simulink model "BF_analyse"  (R2021b)
settings: Solver=VariableStepAuto  StartTime=0.0  StopTime=10.0  RelTol=1e-3
values from neighbouring files (symbols this model uses):
  A = [0 0 0  1 0 0   0 0 0   0 0 0 ... (first row only)    [systune_gain_scheduling.m]    (also in systune_variable_gain_scheduling_LPV.m)
  B = [0 0 0 0 ... (first row only)    [systune_gain_scheduling.m]    (also in systune_variable_gain_scheduling_LPV.m)
  B2 = [0 0 ... (first row only)    [systune_gain_scheduling.m]    (also in systune_variable_gain_scheduling_LPV.m)
  C = eye(12)    [systune_gain_scheduling.m]    (also in systune_variable_gain_scheduling_LPV.m)
  C_control = [1 0 0 0 0 0 0 0 0 1 0 0 ... (96 elements, 8x12)]    [matrix_systune.mat]    (also in systune_gain_scheduling.m = [C(1:7,:);C(9,:)]; systune_variable_gain_scheduling_LPV.m = [C(1:7,:);C(9:12,:)])
  D = zeros(12,6)    [systune_gain_scheduling.m]    (also in systune_variable_gain_scheduling_LPV.m)
  F = [1  0; 1  0; 0  1; 0  1]    [matrix_systune.mat]    (also in systune_gain_scheduling.m = [1 0; 1 0; 0 1; 0 1]; systune_variable_gain_scheduling_LPV.m = [1 0; 1 0; 0 1; 0 1])
  H_val = [-3.93459642094 -3.24554713181 -2.11327628336 -1.80855211908 3.43219949722 2.62084214256 -1.92032774197 -0.213602899472 -0.287812339562 -2.02272198404 12.6924277468 7.31949494852 ... (16 elements, 2x8)]    [matrix_systune.mat]    (also in systune_gain_scheduling.m = H_val.D; systune_variable_gain_scheduling_LPV.m = getBlockValue(T,'H'))
  K_val = [1.47198665157 4.470210116 3.61413916963 0.604491366688 0.55127309979 2.66067735588 2.04948356431 0.425094627773 -2.02824390874 -3.0806217076 -2.7864483599 -0.205582925416 ... (32 elements, 4x8)]    [matrix_systune.mat]    (also in systune_gain_scheduling.m = K_val.D; systune_variable_gain_scheduling_LPV.m = getBlockValue(T,'K'))
  x_12 = [[0; 0; 0]; [0; 0; 0]; [0; sin(angle/2); 0]; [0; 0; 0]]    [systune_gain_scheduling.m]    (also in systune_variable_gain_scheduling_LPV.m)
settings Model: Creator=florian  LastModifiedBy=florian

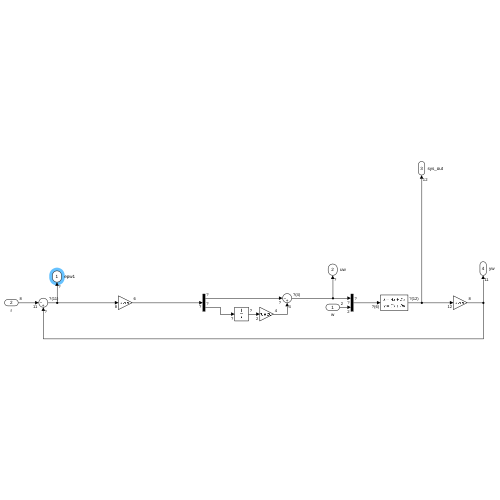
[thumbnail: Simulink's stored preview of the top-level diagram]
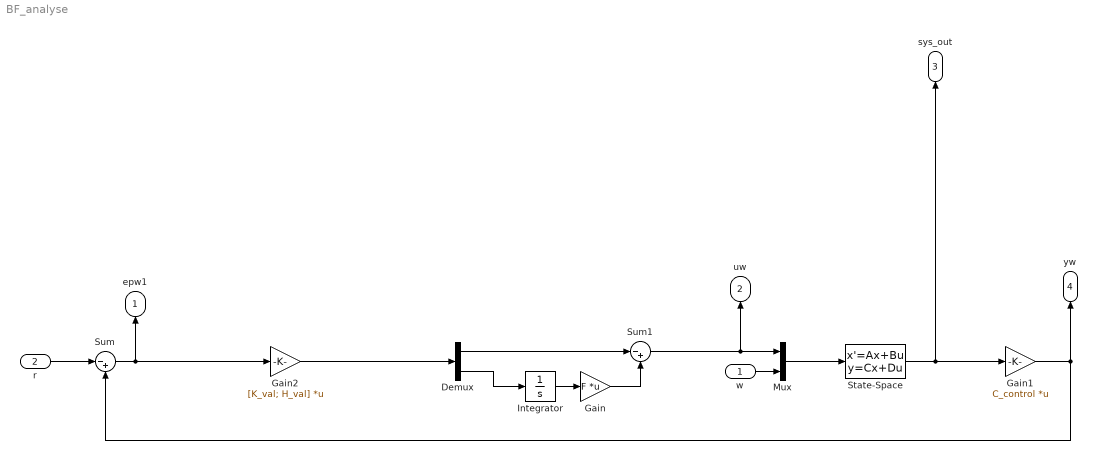
== system BF_analyse ==
  w : Inport  PortDimensions=2
  r : Inport  Port=2  PortDimensions=8
  Demux : Demux  Outputs=2
  Gain : Gain  Gain=F  Multiplication=Matrix(K*u) (u vector)
  Gain1 : Gain  Gain=C_control  Multiplication=Matrix(K*u) (u vector)
  Gain2 : Gain  Gain=[K_val; H_val]  Multiplication=Matrix(K*u) (u vector)
  Integrator : Integrator
  Mux : Mux  Inputs=2
  State-Space : StateSpace  A=A  B=[B, B2]  C=C  D=D  InitialCondition=x_12
  Sum : Sum  Inputs=|-+
  Sum1 : Sum  Inputs=|-+
  epw1 : Outport  InitialOutput=0
  uw : Outport  Port=2  InitialOutput=0
  sys_out : Outport  Port=3  PortDimensions=12
  yw : Outport  Port=4
  wires:
  Demux/2 -> Integrator/1
  Sum1/1 -> uw/1, Mux/1
  Sum/1 -> Gain2/1, epw1/1
  Gain2/1 -> Demux/1
  State-Space/1 -> Gain1/1, sys_out/1
  Gain/1 -> Sum1/2
  w/1 -> Mux/2
  Gain1/1 -> yw/1, Sum/2
  Demux/1 -> Sum1/1
  Mux/1 -> State-Space/1
  r/1 -> Sum/1
  Integrator/1 -> Gain/1
